simulink model "modelul2cerinta7"  (R2022b)
settings: Solver=VariableStepAuto  StartTime=0.0  StopTime=30  RelTol=1e-3
undefined symbols (not defined in the file or in its folder): par
settings Model: Creator=zuch3e  LastModifiedBy=zuch3e
settings DataIOCC: ReturnWorkspaceOutputs=off

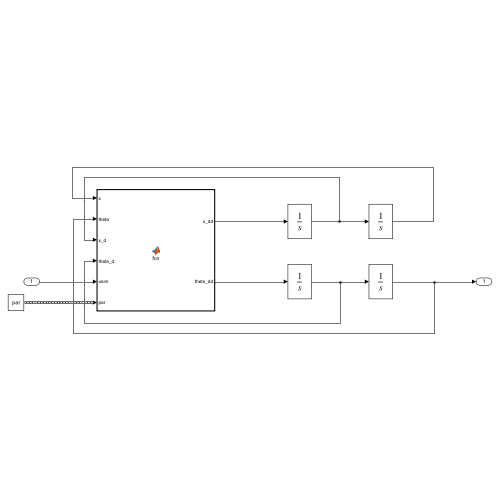
[thumbnail: Simulink's stored preview of the top-level diagram]
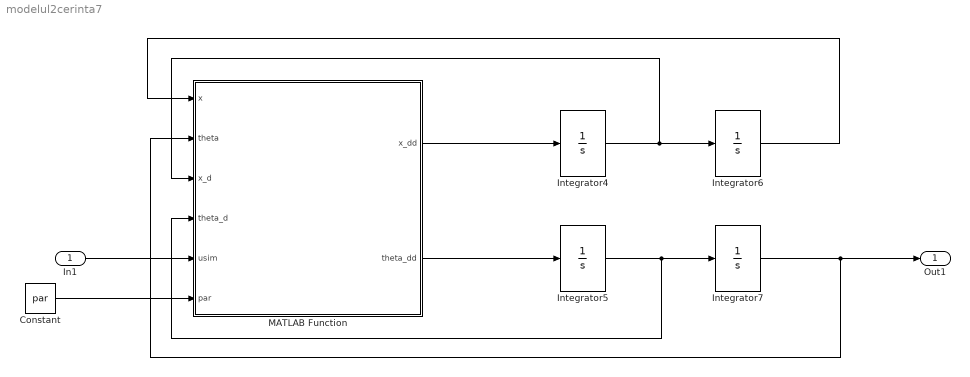
== system modelul2cerinta7 ==
  In1 : Inport
  Constant : Constant  Value=par  OutDataTypeStr=Bus: par_bus
  Integrator{4..7} (4 alike) : Integrator
  MATLAB Function : MATLAB Function  TreatAsAtomicUnit=on
  Out1 : Outport
  wires:
  MATLAB Function/1(x_dd) -> Integrator4/1
  Integrator4/1 -> MATLAB Function/3(x_d), Integrator6/1
  Integrator6/1 -> MATLAB Function/1(x)
  Integrator7/1 -> Out1/1, MATLAB Function/2(theta)
  Integrator5/1 -> MATLAB Function/4(theta_d), Integrator7/1
  MATLAB Function/2(theta_dd) -> Integrator5/1
  Constant/1 -> MATLAB Function/6(par)
  In1/1 -> MATLAB Function/5(usim)

== matlab function modelul2cerinta7/MATLAB Function ==
  data: x input; x_dd output; theta input; x_d input; theta_d input; usim input; par input; theta_dd output
function [x_dd, theta_dd] = fcn(x,theta,x_d,theta_d,usim, par)
x_dd = ((par.l0 + x) * (theta_d^2)) - (par.k*x)/par.m + par.g*cos(theta) - par.zeta*x_d;
theta_dd = ((-1)*par.g*sin(theta))/(par.l0 + x) - (2*x_d*theta_d)/(par.l0 + x) - par.zeta*theta_d + usim/(par.m*((par.l0 + x)^2));
end
